simulink model "task1b"  (Simulink 7.5)
settings: Solver=ode45  StartTime=2.0  StopTime=10.0  RelTol=1e-3
settings Model: Creator=Dranik_win  LastModifiedBy=Dranik_win

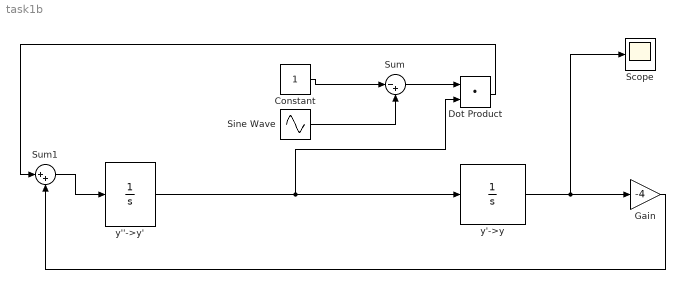
== system task1b ==
  Constant : Constant  OutDataType=fixdt(1, 16)  OutScaling=2^0
  Dot Product : DotProduct  OutDataType=fixdt(1, 16)  OutScaling=2^-10  InputSameDT=on  OutDataTypeStr=Inherit: Inherit via internal rule
  Gain : Gain  Gain=-4  ParameterDataType=fixdt(1, 16)  ParameterScaling=2^0  OutDataType=fixdt(1, 16)  OutScaling=2^0
  Scope : Scope
  Sine Wave : Sin  Amplitude=1  Bias=0  Frequency=1  Phase=pi/2  Samples=10  SampleTime=0  Offset=0
  Sum : Sum  Inputs=|-+  OutDataType=fixdt(1, 16)  OutScaling=2^0
  Sum1 : Sum  Inputs=|++  OutDataType=fixdt(1, 16)  OutScaling=2^0
  y''->y' : Integrator  InitialCondition=1
  y'->y : Integrator  InitialCondition=-1
  wires:
  y''->y'/1 -> Dot Product/2, y'->y/1
  Sum/1 -> Dot Product/1
  Sine Wave/1 -> Sum/2
  Constant/1 -> Sum/1
  Dot Product/1 -> Sum1/1
  y'->y/1 -> Gain/1, Scope/1
  Gain/1 -> Sum1/2
  Sum1/1 -> y''->y'/1
